simulink model "mOvertakeManeuver"  (R2018b)
settings: Solver=VariableStepAuto  StartTime=0.0  StopTime=simTime  RelTol=1e-3
PreLoadFcn:
  | load 'tableStructure.mat'
InitFcn:
  | modelParams
  | clear markedSmartActorCount;
values from neighbouring files (symbols this model uses):
  initYPos = (scene.RoadNetwork.RoadCenters(1, 2) - laneWidth / 2)    [modelParams.m]
  initYPosRogue = (scene.RoadNetwork.RoadCenters(1, 2) - laneWidth / 2)    [modelParams.m]
  laneWidth = roadWidth / (scene.RoadNetwork.NumMarkings - 1)    [modelParams.m]
  maxLanes = 10    [modelParams.m]
  maxVehicles = 25    [modelParams.m]
  minOvertakeProximity = 50    [modelParams.m]
  numActors = length(scene.vehiclePoses(1).ActorPoses)    [modelParams.m]    (also in sessionLogReader.m = numel(inStruct); visualizer.m = numel(actors))
  numAddedRogueActors = 0    [modelParams.m]
  numLanes = scene.RoadNetwork.NumLanes    [modelParams.m]    (also in sessionLogReader.m = numMarkings-1)
  numSmartActors = 0    [modelParams.m]
  numSmartActorsDM = 0    [modelParams.m]
  rogueActorIdBase = 4000    [modelParams.m]
  safeTimeGap = 1.4    [modelParams.m]
  sensorRange = 600    [modelParams.m]
  smartActors = 0    [modelParams.m]    (also in sessionLogReader.m = repmat(actorPoses(1), [obj.NumSmartActors, 1]))
  smartActorsDM = 0    [modelParams.m]    (also in sessionLogReader.m = repmat(actorPoses(1), [obj.NumSmartActorsDM, 1]))
  standStillGap = 10    [modelParams.m]
  W_SPEC = [Ln1;vdes;vmax;AXadd;AXmult;BXadd;BXmult;EXadd;EXmult;CXconst;CXadd;CXmult;OPDVmult;OPDVadd;BNULLmult;BMAXmult;FAKTORVmult;BMINadd;BMINmult;      RND1n;RND2n;RND3n;RND4n;NRND]    [wiedemannParams.m]
undefined symbols (not defined in the file or in its folder): actorPoseInit, addedRogueVelocity, addedRogueXPosition, DiscIntNeverNeededParam
libraries: dataTableBlockslib x2, mpcadaslib x1
(part 2 of 3)

== matlab function mOvertakeManeuver/Wiedemann-74 Driver Model/Apply driver-model/Extract InitPos and InitVel Vector ==
  data: accelVector input; smartActorsDM parameter; accelVector output; initVelVector output; initPosVector output; actorPoseInit parameter
function [accelVector, initVelVector, initPosVector] = extractInitPoses(accelVector, smartActorsDM, actorPoseInit)
% Extract init poses for vehicles with car-following model.
numActors = length(smartActorsDM);
initPosVector = ones(numActors,1);
initVelVector = ones(numActors,1);
for i = 1 : numActors
    initPosVector(i) = actorPoseInit(uint32(smartActorsDM(i))).Position(1);
    initVelVector(i) = actorPoseInit(uint32(smartActorsDM(i))).Velocity(1);
    if actorPoseInit(uint32(smartActorsDM(i))).Yaw == 180 % Actor is moving in negative - x dir
        accelVector(i) = -accelVector(i);
    end
end

== matlab function mOvertakeManeuver/Wiedemann-74 Driver Model/Apply driver-model/Wiedemann-driver-model/Judgement/Wiedemann74 ==
  data: xn input; bn output; vn input; xn1 input; vn1 input; bn1 input; regime output; AXAdd parameter; BXMult parameter; W_SPEC input; maxAccel parameter; maxDecel parameter; vMax parameter; vDes parameter
function [bn,regime] = wiedemann74(xn, vn, xn1, vn1, bn1, AXAdd, BXMult, W_SPEC, maxAccel, maxDecel, vMax, vDes)
% Wiedemann 74 car-following model
% input
% xn: ego vehicle position
% vn: ego vehicle velocity
% xn1: lead vehicle position
% vn1: lead vehicle velocity
% bn1: lead vehicle acceleration
% W_SPEC: model parameters
% output
% bn: ego vehicle acceleration command, i.e., driver's judgement
% regime: driver's operating mode
% (1 = following, 2 = free driving, 3 = approaching, 4 = emergency, -1 = danger)

numActors = size(xn, 1);
persistent dirAccel dx_old dv_old
if isempty(dirAccel)
    dirAccel = ones(numActors, 1);
end
if isempty(dx_old)
    dx_old = ones(numActors, 1);
    for i = 1 : numActors
        dx_old(i) = abs(xn1(i) - xn(i));
    end
end
if isempty(dv_old)
    dv_old = ones(numActors, 1);
    for i = 1 : numActors
        dv_old(i) = vn(i) - vn1(i);
    end
end

bn = ones(numActors, 1);
regime = ones(numActors, 1);
for i = 1 : numActors
    % variables
    dx = abs(xn1(i) - xn(i)); % [m] space headway
    dv = vn(i) - vn1(i); % [m/s] difference in speed
    % parameters
    % User-configured parameters
    AXadd = AXAdd(i);
    BXmult = BXMult(i);
    vmax = vMax(i);
    vdes = vDes(i);
    % Other parameters for which all the cars share the same value
    Ln1 = W_SPEC(1);
    AXmult = W_SPEC(5);
    BXadd = W_SPEC(6);
    EXadd = W_SPEC(8);
    EXmult = W_SPEC(9);
    CXconst = W_SPEC(10);
    CXadd = W_SPEC(11);
    CXmult = W_SPEC(12);
    OPDVmult = W_SPEC(13);
    OPDVadd = W_SPEC(14);
    BNULLmult = W_SPEC(15);
    BMAXmult = 3.5 / vmax;
    FAKTORVmult = W_SPEC(17);
    BMINadd = W_SPEC(18);
    BMINmult =  1.5 / vmax;
    RND1n = W_SPEC(20);
    RND2n = W_SPEC(21);
    RND3n = W_SPEC(22);
    RND4n = W_SPEC(23);
    NRND = W_SPEC(24);
    
    % threshold of driver's operating regime
    % AX: Minimum distance headway (front-bumper to front-bumper distance) in a standstill condition
    AX = Ln1 + AXadd + AXmult * RND1n;
    
    % ABX: Minimum desired following distance
    v_slower = min(vn(i), vn1(i));
    BX = (BXadd + BXmult * RND1n) * sqrt(v_slower);
    ABX = AX + BX;
    
    % SDX: Maximum desired following distance
    EX = EXadd + EXmult * (NRND - RND2n);
    SDX = AX + EX * BX;
    
    % SDV: Threshold at which driver recognizes that he is approaching a slower vehicle
    CX = CXconst * (CXadd + CXmult * (RND1n + RND2n));
    SDV = ((dx - Ln1 - AX) / CX)^2;
    
    % CLDV: Threshold for speed difference in a closing process during a following condition
    CLDV = SDV; % CLDV is assumed to be equal to SDV
    
    % OPDV: Threshold for speed difference in an opening process during a following condition
    OPDV = CLDV * (-OPDVadd - OPDVmult * NRND);
    
    % acceleration/deceleration command
    if (dx >= ABX) && (dv >= OPDV) && (dx <= SDX) && (dv <= SDV) % following
        if (SDV < dv_old(i)) || (dx_old(i) < ABX) % passing SDV, ABX
            dirAccel(i) = -1;
        elseif (dv_old(i) < OPDV) || (SDX < dx_old(i)) % passing OPDV, SDX
            dirAccel(i) = 1;
        end
        bnull = BNULLmult * (RND4n + NRND);
        bn(i) = dirAccel(i) * bnull;
        regime(i) = 1;
    elseif ((dx > ABX) && (dv < OPDV)) || ((dx > SDX) && (dv < SDV)) % free driving
        FaktorV = vmax / (vdes + FAKTORVmult * (vmax - vdes));
        bmax = BMAXmult * (vmax - v_slower * FaktorV);
        bn(i) = bmax;
        regime(i) = 2;
    elseif (dv > SDV) && (dx > ABX) % approaching
        bn(i) = 0.5 * dv^2 / (ABX - (dx - Ln1)) + bn1(i);
        regime(i) = 3;
    elseif (dx > AX) && (dx < ABX) % emergency
        bmin = -BMINadd - BMINmult * RND3n + BMINmult * vn(i);
        bn(i) = 0.5 * dv^2 / (ABX - (dx - Ln1)) + bn1(i) + bmin * (ABX - (dx - Ln1)) / BX;
        regime(i) = 4;
    else % danger
        bn(i) = 0;
        regime(i) = -1;
    end
    
    if(bn(i) > maxAccel(i)) % Limiting output accel/decel by upper and lower bounds
        bn(i) = maxAccel(i);
    elseif(bn(i) < maxDecel(i))
        bn(i) = maxDecel(i);
    end
    
    if(bn(i) < 0 && vn(i) < 0) % Not allowing backward-movement
        bn(i) = 0;
    end
    
    dv_old(i) = dv;
    dx_old(i) = dx;
end

== matlab function mOvertakeManeuver/Wiedemann-74 Driver Model/Get Follow and Lead car ==
  data: follPos output; follVel output; leadPos output double; leadVel output double; smartActorsDM parameter; leadAcc output; sensorRange parameter; timestamp input
function [follPos, follVel, leadPos, leadVel, leadAcc] = extractFollowAndLeadCar(...
    smartActorsDM, sensorRange, timestamp)
% For the cars with driver model, extract their info as well as their
% respective lead car info from the data-table.

% To store the current timestamp and velocity of respective
% lead vehicles for calculation of their acceleration in the next step.
% Also, as acceleration calculation requires velocity at two timestamps,
% 3rd column in this information has the flag indicating whether previous
% velocity info is available.
persistent prevInfo;
if(isempty(prevInfo))
    prevInfo = zeros(length(smartActorsDM), 3);
end

leadPos = ones(length(smartActorsDM), 1);
leadVel = ones(length(smartActorsDM), 1);
follPos = ones(length(smartActorsDM), 1);
follVel = ones(length(smartActorsDM), 1);
leadAcc = zeros(length(smartActorsDM), 1);

for i = 1 : length(smartActorsDM)
    key = getActorTableEntryKey(uint32(1), smartActorsDM(i));
    if(key ~= -1) % If an entry exist
        smartVehInfo = getActorTableEntry(key);
        [numVehAhead, vehiclesAheadInfo] = getVehAheadSorted(key);
        if(numVehAhead == 0)
            % There is no vehicle ahead of this smart vehicle
            % Give impression that vehicle ahead is out of sensor range
            if smartVehInfo.Velocity(1) < 0
                leadPos(i) = smartVehInfo.Position(1) - sensorRange;
            else
                leadPos(i) = smartVehInfo.Position(1) + sensorRange;
            end
            leadVel(i) = smartVehInfo.Velocity(1);
            leadAcc(i) = 0;
            prevInfo(i, 3) = 0;
        else
            leadPos(i) = vehiclesAheadInfo(1).Position(1); % Get position of vehicle just ahead.
            leadVel(i) = vehiclesAheadInfo(1).Velocity(1); % Get speed of vehicle just ahead.
            if(prevInfo(i, 3) == 1) % If previous velocity known for accel calculation
                leadAcc(i) = (vehiclesAheadInfo(1).Velocity(1) - prevInfo(i, 2)) / ...
                    (timestamp - prevInfo(i, 1));
            else
                leadAcc(i) = 0 ;
            end
        end
        follPos(i) = smartVehInfo.Position(1);
        follVel(i) = smartVehInfo.Velocity(1);
        prevInfo(i, 1) = timestamp;
        prevInfo(i, 2) = vehiclesAheadInfo(1).Velocity(1);
        prevInfo(i, 3) = 1; % Acceleration can be calculated at next time-step.
        leadVel(i) = abs(leadVel(i));
        follVel(i) = abs(follVel(i));
        if smartVehInfo.Yaw == 180 % Actor is moving in negative - x dir
            leadAcc(i) = -leadAcc(i);
        end
    end
end

== matlab function mOvertakeManeuver/Services/Find approaching vehicles in the left lane/MATLAB Function ==
  data: refPose input; matched output; candidatePose input; sensorRange parameter; laneWidth parameter; numLanes parameter
function matched = findVehiclesAheadLeftLane(refPose, candidatePose, sensorRange, laneWidth, numLanes)
% For any vehicle, get the vehicles ahead in the opposite lane. Query is
% assumed to called for a vehicle moving in +ve x-direction.
% refVeh - Query-Calling vehicle
% candidateVeh - Actor to be processed as candidate for matching the criteria.

laneBoundaries = zeros(1, numLanes + 1);
% Getting the key corresponding to the actorId from data-table
key = getScenarioTableEntryKey(uint32(1), refPose.ActorID);
completeLaneBoundaryInfo = getScenarioTableEntry(key);
for i = 1 : size(laneBoundaries, 2)
    laneBoundaries(1, i) = completeLaneBoundaryInfo.coordinates(i, 2);
end
laneIndx = -1;
% Find own lane information based on lane boundary info and own pose info.
for i = 1 : size(laneBoundaries, 2) - 1
    if (refPose.Position(2) <= laneBoundaries(1, i) && refPose.Position(2) >= laneBoundaries(1, (i + 1)))
        laneIndx = i;
        break;
    end
end
if laneIndx < 0
    matched = false;
elseif laneIndx <= numLanes
    xGap = (candidatePose.Position(1) - refPose.Position(1));
    yGap = (candidatePose.Position(2) - refPose.Position(2));
    gap = sqrt(xGap * xGap + yGap * yGap);
    
    % Candidate actor must be ahead AND in Range AND In opposite(left) lane
    if ((xGap > 0)  && gap < sensorRange && ((candidatePose.Position(2) >= laneBoundaries(1, laneIndx))) ...
            && ((candidatePose.Position(2) <= (laneBoundaries(1, laneIndx) +  laneWidth))))
        matched = true;
    else
        matched = false;
    end
else
    matched = false;
end

== matlab function mOvertakeManeuver/Scene Management/Publish To Data Table/update data tables ==
  data: actors input; laneBoundaryInfo input; maxLanes parameter; smartActorsDM parameter; smartActors parameter
function updateDataTables(actors, laneBoundaryInfo, maxLanes, smartActorsDM, smartActors)
% Write into actor-pose table and scene table(containing lane boundary information)

% Write into actor-pose table
for k = 1 : length(actors)
    % Write the actor-poses into the data-table (Except for the smart
    % actors to avoid re-writing in the data-table the same data which we just read)
    if ~(ismember(actors(k).ActorID, smartActors) || ismember(actors(k).ActorID, smartActorsDM))
        setActorTableEntry(actors(k).ActorID, actors(k)); % Use key to update the row entry.
    end
end

% Write lane boundary information of smart actors into scene data-table.
numLanes = laneBoundaryInfo.NumLaneBoundaries;
for i = 1 : length(laneBoundaryInfo.ActorIDs)
    laneBoundary.ActorID = laneBoundaryInfo.ActorIDs(i);
    laneBoundary.coordinates = ones(maxLanes, 3) * (double(intmax('uint32')));
    for j = 1 : numLanes % For each lane writing x,y,z coordinates
        for k = 1 : 3 % For x,y and z
            laneBoundary.coordinates(j, k) = laneBoundaryInfo.LaneBoundaries(i, j).Coordinates(1, k);
        end
    end
    setScenarioTableEntry(laneBoundary.ActorID, laneBoundary); % Write into scene data-table.
end

== stateflow chart mOvertakeManeuver/Smart Actor/Smart Actor system/Planner/Plan Library and its evaluation/Plan 1/Plan 1: Overtake Maneuver/checkOvertakeFeasibility/Check feasibilty of the overtake ==
  note: Algorithm to decide if in the current environment, smart-car can start an overtake-maneuver right away.
      | It does so by anticipating movement of other vehicles and its own trajectory for overtake maneuver.
      |
      | Note: The overtake maneuver plan assumes that all other actors move straight with constant speed.
      |
      | Structure of this chart is such, that it sequentially does various checks for ensuring that overtake mauver is safe.Whenever any check fails the overtake is deemed as unsafe. Only when all the conditions meet, the chart returns 'overtakeDecision=1' (which happens at the bottom-right of chart after passing all the tests).
  (default) -> (junction 615) : {
      | actorStruct = struct('ActorID',double(intmax('uint32')), 'Position', [0 0 0], ...
      |                       'Velocity', [0 0 0], 'Roll', 0, 'Pitch', 0, 'Yaw', 0, ...
      |                       'AngularVelocity', [0 0 0]);
      |
      | % Variables initialization
      | vehiclesAheadList = repmat(actorStruct, maxVehicles, 1);
      | rogueOppDir  = repmat(actorStruct, maxVehicles, 1);
      | overtakeDecision = 0;
      | t1 = 0;  % Time spent for moving towards opposite direction lane.
      | t2 = 0;  % Time spent for moving in opposite direction lane.
      | t3 = 0;  % Time spent for merging back into original lane
      |
      | % Value = 1 if smart vehicle is going to merge between 2 vehicles after overtake.
      | % Value = 0 if smart vehicle would not have a vehicle ahead after overtake.
      | mergeBehindVehFlag = 0;
      |
      | leftLaneCenter = getLeftLane(currPose);
      | precedVehInfo = actorStruct;
      | }
  (junction 615) -> (junction 616) [order 1] : % If left lane present
      | [leftLaneCenter ~= realmax('double') ]
  (junction 615) -> (junction 660) [order 2] : {
      | % No lane on the left where smart-vehicle
      | % can move temporarily for overtake
      | overtakeDecision = 0;
      | }
  (junction 616) -> (junction 713) : {
      | leftLaneChangeDistY = leftLaneCenter - currPose.Position(2);
      |  % Assuming 45 deg movement towards adjacent lane
      | leftLaneChangeDistance =  leftLaneChangeDistY * 1.414;
      | rightLaneChangeDistance  = laneWidth * 1.414;
      | smartActorPosition = currPose.Position;
      |
      | % Get list of vehicles ahead moving in the same lane in sorted
      | % order of their distance from smart vehicle.
      | [count, vehiclesAheadList] = getVehAheadSameLaneSorted(currPose);
      |
      | % Set the limit on number of vehicles allowed to be overtaken
      | % in a single go based on driver aggresiveness level.
      | maxOvertakeCapability =  aggressivenessLevel;
      | i=1;
      | }
  (junction 713) -> (junction 709) [order 1] : [i<=count]
  (junction 710) -> (junction 713) : {
      |      i=i+1;
      | }
  (junction 713) -> (junction 467) [order 2]
  (junction 709) -> (junction 710) : {
      |     % Convert to self-centered pose
      |      vehiclesAheadList(i) = ...
      |      globalToSelfCentered(currPose, vehiclesAheadList(i));
      | }
  (junction 467) -> (junction 660) [order 2] : {
      | % No vehicle ahead to overtake
      | overtakeDecision = 0;
      | }
  (junction 467) -> (junction 469) [order 1] : [count > 0  ]
  (junction 660) -> (junction 663)
  (junction 469) -> (junction 471) : {
      | % Get vehicle just ahead
      | nearestVehInfo = vehiclesAheadList(1);
      | }
  (junction 471) -> (junction 663) [order 2] : {
      | % Vehicle ahead is too far so no need to overtake
      | overtakeDecision = 0;
      | }
  (junction 471) -> (junction 473) [order 1] : % Vehicle ahead must be close enough
      | % to initiate overtake
      |   [nearestVehInfo.Position(1) < ...
      |    minOvertakeProximity]
  (junction 663) -> (junction 666)
  (junction 473) -> (junction 27)
  (junction 27) -> (junction 47) [order 1] : [count < maxOvertakeCapability]
  (junction 27) -> (junction 48) [order 2] : {
      |      overtakeLen = maxOvertakeCapability;
      | }
  (junction 47) -> (junction 49) : {
      |     overtakeLen = count ;
      | }
  (junction 49) -> (junction 48)
  (junction 48) -> (junction 70)
  (junction 70) -> (junction 666) [order 2] : {
      | % No possibility of overtake-maneuver.
      | % All possibilities right from max-capability
      | % overtake to 1-vehicle-overtake are checked
      | % but none was feasible.
      | overtakeDecision = 0;
      | }
  (junction 70) -> (junction 69) [order 1] : % Loop through all possible overtake maneuvers.
      | %Start feasibilty check from maximum length overtake upto 1-vehicle-overtake
      | % and exit the loop whenever first feasibility check is successful
      | [overtakeLen > 0]
  (junction 666) -> (junction 264)
  (junction 682) -> (junction 70) : {
      | % Decrement for 1-lesser level overtake
      | overtakeLen = overtakeLen - 1;
      | }
  (junction 69) -> (junction 621) : {
      |     % Vehicle to be checked for overtaking
      |     followVehInfo = vehiclesAheadList(overtakeLen);
      | }
  (junction 621) -> (junction 682) [order 2] : % Cannot overtake a vehicle moving
      | % at a higher speed than this (smart) vehicle's
      | % max speed.
      | % Check for 1-lesser level overtake
  (junction 621) -> (junction 73) [order 1] : % Overtake possible only if vehicle ahead is moving at
      |  % lesser speed than smart actor's max speed.
      |  [maxVelocity >  ...
      | (followVehInfo.Velocity(1) + currPose.Velocity(1)) ...
      | && currPose.Velocity(1) > 0]
  (junction 73) -> (junction 81) [order 1] : [overtakeLen < count]
  (junction 685) -> (junction 682)
  (junction 73) -> (junction 96) [order 2]
  (junction 81) -> (junction 92) : {      % Vehicle Id to be checked for merging behind
      |         % Smart vehicle is cheking possiblity of merging between actors
      |         % having pose 'followVehInfo' and 'precedVehInfo'
      |         mergeBehindVehFlag = 1;
      | 	  precedVehInfo = vehiclesAheadList(overtakeLen + 1);
      |         reqSafeGap = 2 * ((currPose.Velocity(1) + precedVehInfo.Velocity(1)) ...
      |                                * safeTimeGap + standStillGap);
      |         gap = precedVehInfo.Position(1) - followVehInfo.Position(1);
      | }
  (junction 92) -> (junction 685) [order 2] : % Not enough gap present between two vehicles
      | % for merging in between after overtake maneuver
      | % Check for 1-lesser level overtake
  (junction 92) -> (junction 93) [order 1] : % Not enough gap between vehicles in smart actor's
      | % lane to merge in between after overtaking.
      | [gap >= reqSafeGap]
  (junction 669) -> (junction 685)
  (junction 93) -> (junction 94)
  (junction 94) -> (junction 96)
  (junction 96) -> (junction 608) : {
      |     [t1, smartVehXT1, t2, smartVehXT2, t3, smartVehXT3, smartVehSpeedT3] =  ...
      |     anticipateManeuverSubTrajectories();
      |
      |     T = t1 + t2 +t3; % Total time taken for overtake maneuver
      |     }
  (junction 608) -> (junction 483) : {
      |    % Need to check safety w.r.t vehicle coming from opposite direction
      |     oppositeDirSafety = anticipateOppositeDirTrafficSafety();
      | }
  (junction 483) -> (junction 669) [order 2] : % Not safe w.r.t oppsite direction traffic
      | % Check for 1-lesser level overtake
  (junction 483) -> (junction 185) [order 1] : [oppositeDirSafety==1]
  (junction 678) -> (junction 669)
  (junction 185) -> (junction 245) : {
      |     isSafeAfterOvertake =  ...
      |     anticipateSafetyAfterManeuverCompletion(smartVehXT3);
      | }
  (junction 245) -> (junction 678) [order 2] : %  Not safe w.r.t. to vehicles it is planning
      | % to merge in between after overtake.
      | % Check for 1-lesser level overtake
  (junction 245) -> (junction 672) [order 1] : [isSafeAfterOvertake==1]
  (junction 672) -> (junction 192)
  (junction 192) -> (junction 264) : {
      | % All conditions met for safe overtake.
      | overtakeDecision = 1;
      | }
  (junction 264) -> (junction 688)
  data: time1 function_output; smartXPos1 function_output; time2 function_output; smartXPos2 function_output; time3 function_output; smartXPos3 function_output; smartXVel3 function_output; isSafe function_output; isSafe function_output; smartXPosT3 function_input; overtakeDecision output; currPose input Bus: Vehicle; maxVelocity parameter; maxAcceleration parameter; nearestVehInfo local Bus: Vehicle; safeTimeGap parameter; standStillGap parameter; followVehXT2 local; followVehspeedT2 local; leftLaneChangeDistY local; rightLaneChangeDistance local; T local; a local; b local; c local; count local; d local; smartActorPosition local; smartVehXT1 local; smartVehXT2 local; followVehSpeed local; followVehXT1 local; gap local; gapBack local =0; gapFront local =0; leadRogueOppDirInfo local Bus: Vehicle; leadRogueOppDirPos local =0; leftLaneChangeDistance local; mergeBehindVehFlag local; oppRogueCount local; overtakeLen local; reqSafeGap local; reqSafeGapBack local =0; reqSafeGapFront local =0; rogueOppDir local Bus: Vehicle; s2 local; s21 local; t21 local; t22 local; vehiclesAheadList local Bus: Vehicle; smartVehSpeedT3 local; followVehXT3 local =0; smartVehXT3 local; pPrecedingRogue local =0; vehicleAheadOvertakenRogueDetails local Bus: Vehicle; laneWidth parameter; actorStruct local Bus: Vehicle; maxOvertakeCapability local; precedVehInfo local Bus: Vehicle; followVehInfo local Bus: Vehicle; i local; t1 local; t3 local; t2 output; d1 local; d2 local; t23 local; safeGapDeficit local; maxVehicles parameter; minOvertakeProximity parameter; leftLaneCenter local; oppositeDirSafety local; isSafeAfterOvertake local; aggressivenessLevel parameter
  function [time1, smartXPos1, time2, smartXPos2, time3, smartXPos3, smartXVel3] = anticipateManeuverSubTrajectories:
    | function [time1, smartXPos1, time2, smartXPos2, time3, smartXPos3, smartXVel3] = anticipateManeuverSubTrajectories()
    | % Anticipate smart-actors sub-trajectories for overtake-maneuver trajectory.
    | % time1 - Time soent in sub-trajectory 1 ( i.e. Movement towards left lane)
    | % smartXPos1 - Smart actor's X-pos at the end of sub-trajectory 1
    | % time2 - Time soent in sub-trajectory 2 ( i.e. Movement on the left lane)
    | % smartXPos2 - Smart actor's X-pos at the end of sub-trajectory 2
    | % time3 - Time soent in sub-trajectory 3 ( i.e. Movement back to original lane)
    | % smartXPos3 - Smart actor's X-pos at the end of sub-trajectory 3
    | % smartXVel3 - Smart actor's X-vel at the end of sub-trajectory 3
    | 
    | % Calculate the time to reach the adjacent lane
    | time1 = leftLaneChangeDistance / currPose.Velocity(1) ;
    | 
    | % Anticipated position and velocity of smart Veh and 'followVehId' after
    | % 'time1' time units after overtake maneuver start i.e the time after which
    | % smart vehicle reaches the adjacent lane.
    | % Note: This is just anticipated information. Vehicles move in real only if
    | % overtake maneuver turn out to be safe in the logic below.
    | smartXPos1 =   currPose.Position(1) + leftLaneChangeDistance;
    | followVehXT1 =  (currPose.Position(1) + followVehInfo.Position(1)) + ...
    |     (currPose.Velocity(1) + followVehInfo.Velocity(1)) * time1;
    | smartVehSpeedT1 = currPose.Velocity(1);
    | followVehSpeed = currPose.Velocity(1) + followVehInfo.Velocity(1);
    | 
    | % Anticipitation of position and velocity info after t = time1+time2.
    | % 'time2' is the time elapsed from the point smart vehicle reached adjacent
    | % lane upto the time after which smart vehicle has accumulated safe gap with
    | % respect to the vehicle to be overtaken while moving parallel to it in the
    | % adjacent lane. This condition when used with Newton's equations of motion
    | % results into a quadratic equation of form ax2+bx+c where x='time2' and
    | % a,b,c defined below.
    | a = 0.5 * maxAcceleration;
    | b = smartVehSpeedT1 - followVehSpeed;
    | c = smartXPos1 - followVehXT1 - followVehSpeed * safeTimeGap - standStillGap;
    | d = (b ^ 2) - (4 * a * c);
    | time2a = (- b + sqrt(d)) / (2 * a); % first root of equation
    | time2b = (- b - sqrt(d)) / (2 * a); % second root of equation
    | if(time2a > 0) % Only positive root is meaningful
    |     time2 = time2a;
    | else
    |     time2 = time2b;
    | end
    | 
    | smartVehSpeedT2 = smartVehSpeedT1 + maxAcceleration * time2; % Speed of smart vehicle after time1 + time2
    | s2 = smartVehSpeedT1 * time2 + 0.5 * maxAcceleration * time2 ^ 2;
    | 
    | if(smartVehSpeedT2 > maxVelocity)
    |     % After time time2 smart vehicle is going to breach
    |     % max velocity allowed, so time time2 is broken into time2a and time2b .
    |     % time2a - time to reach max vel
    |     % time2b - time to accumulate safe gap w.r.t vehicle being overtaken after reaching max velocity
    |     
    |     % Distance travelled in the process of reaching max velocity.
    |     s21 = ((maxVelocity ^ 2) - (smartVehSpeedT1 ^ 2)) / (2 * maxAcceleration);
    |     t21 = (maxVelocity - smartVehSpeedT1) / maxAcceleration;
    |     t22 = ((followVehSpeed * safeTimeGap + standStillGap) - (smartXPos1 + s21) + ...
    |         (followVehXT1 + followVehSpeed * t21)) / (maxVelocity - followVehSpeed);
    |     % Total time travelled by the smart car in adjacent lane to create safeGap between the the rogue car and itself
    |     time2 = t21 + t22;
    |     smartVehSpeedT2 = maxVelocity;
    |     s2 = s21 + maxVelocity * t22 ;
    | end
    | 
    | smartXPos2 = smartXPos1 + s2  ;
    | followVehXT2 = followVehXT1 + followVehSpeed * time2;
    | followVehspeedT2 = followVehSpeed;
    | %total time after which merging into the actual lane will be started
    | T =  time1 + time2 ;
    | 
    | time3 = rightLaneChangeDistance / smartVehSpeedT2;
    | d1 = laneWidth;
    | d2 = followVehspeedT2 * time3;
    | 
    | if(d1 < d2)
    |     safeGapDeficit = d2 - d1;
    |     t23 = safeGapDeficit / (smartVehSpeedT2 - followVehspeedT2);
    |     smartXPos2 = smartXPos2 + smartVehSpeedT2 * t23 ;
    |     followVehXT2 = followVehXT2 + followVehspeedT2 * t23;
    |     T =  T + t23;
    | end
    | 
    | % time3 is the time taken by smart vehicle to again move to its original lane
    | % after it has accumulated safe gap w.r.t to vehicle to be
    | % overtaken. Safety condition at this time is that after merging into the
    | % main lane smart vehicle shouldbe safe wrt the vehicles it is merging
    | % between.
    | 
    | time3 = rightLaneChangeDistance / smartVehSpeedT2;
    | smartXPos3 = smartXPos2 + rightLaneChangeDistance;
    | smartXVel3 = smartVehSpeedT2;
  function isSafe = anticipateOppositeDirTrafficSafety:
    | function isSafe = anticipateOppositeDirTrafficSafety
    | % Anticipate whether smart-actor is safe w.r.t to traffic from opposite
    | % direction for overtake maneuver.
    | 
    | isSafe = 1;
    | % Find the rogue vehicles approaching from the opposite direction
    | [oppRogueCount, rogueOppDir]  = getVehAheadLeftLaneSorted(currPose);
    | for i=1:oppRogueCount % Convert to self-centered pose
    |     rogueOppDir(i) = globalToSelfCentered(currPose, rogueOppDir(i));
    | end
    | i = 1;
    | % For each rogue veh from the opposite direction, check safety.
    | for i = 1 : oppRogueCount
    |     leadRogueOppDirInfo = rogueOppDir(i);
    |     % Its anticipated position after end of subTrajectory-2 i.e after it
    |     % has finished movement on opposite direction lane.
    |     leadRogueOppDirPos = leadRogueOppDirInfo.Position(1) + smartActorPosition(1) ...
    |         + ((leadRogueOppDirInfo.Velocity(1) +  currPose.Velocity(1)) * T);
    |     % Anticipated gap between this and smart vehicle after time = t1 + t2
    |     gap = leadRogueOppDirPos - smartVehXT2 ;
    |     
    |     % Smart actor must not collide or be in unsafe proximity of actor coming from
    |     % opposite direction
    |     if(gap <= 2 * standStillGap)
    |         isSafe = 0; % Not safe
    |         break;
    |     end
    | end
  function isSafe = anticipateSafetyAfterManeuverCompletion (smartXPosT3):
    | function isSafe = anticipateSafetyAfterManeuverCompletion (smartXPosT3)
    | % Anticipate whether smart-actor is safe after it merges back to its original
    | % lane i.e. after completion of overtake maneuver. Basically at that point
    | % smart actor must be safe w.r.t vehicles it is merging in between.
    | 
    | isSafe = 1;
    | followVehSpeed = currPose.Velocity(1) + followVehInfo.Velocity(1);
    | followVehXT1 =  (currPose.Position(1) + followVehInfo.Position(1)) + ...
    |     (currPose.Velocity(1) + followVehInfo.Velocity(1)) * t1;
    | followVehXT2 = followVehXT1 + followVehSpeed * t2;
    | 
    | followVehXT3 = followVehXT2 + followVehSpeed * t3;
    | 
    | vehicleAheadOvertakenRogueDetails = precedVehInfo;
    | reqSafeGapFront =  smartVehSpeedT3  * safeTimeGap + standStillGap;
    | reqSafeGapBack = followVehSpeed * safeTimeGap + standStillGap;
    | pPrecedingRogue = vehicleAheadOvertakenRogueDetails.Position(1) + currPose.Position(1) +  ...
    |     (currPose.Velocity(1) + vehicleAheadOvertakenRogueDetails.Velocity(1)) * T;
    | gapFront =  pPrecedingRogue - smartXPosT3;
    | gapBack =  smartXPosT3 - followVehXT3;
    | 
    | % If there a vehicle ahead after manaeuver then the smart vehicle needs to
    | % check both front and back safety. Otherwise smart vehicle just needs to be
    | % safe with respect to vehicle it is merging ahead of, after overtake.
    | if(mergeBehindVehFlag)
    |     if (gapFront < reqSafeGapFront || gapBack < reqSafeGapBack)
    |         isSafe = 0; % Not safe
    |     end
    | else
    |     if(gapBack < reqSafeGapBack)
    |         isSafe = 0; % Not safe
    |     end
    | end

== matlab function mOvertakeManeuver/Services/Global to self-centered pose conversion/Self-Centered Pose Conversion ==
  data: selfPose input; otherVehPose input Bus: Vehicle; egoCentricInfo output Bus: Vehicle
function egoCentricInfo = globalToSelfCenteredConversion(selfPose, otherVehPose)
% Convert global-coordinate pose of another vehicle to self-centered pose.

egoCentricInfo.ActorID = otherVehPose.ActorID;
egoCentricInfo.Position = otherVehPose.Position - selfPose.Position;
egoCentricInfo.Velocity = otherVehPose.Velocity - selfPose.Velocity;
egoCentricInfo.Roll = otherVehPose.Roll - selfPose.Roll;
egoCentricInfo.Pitch = otherVehPose.Pitch - selfPose.Pitch;
egoCentricInfo.Yaw = otherVehPose.Yaw - selfPose.Yaw;
egoCentricInfo.AngularVelocity = otherVehPose.AngularVelocity - selfPose.AngularVelocity;

== matlab function mOvertakeManeuver/Wiedemann-74 Driver Model/Write smart-actor poses in data-table ==
  data: smartActorsDM parameter; velVector input; posVector input
function updateSmartCarPose(smartActorsDM, velVector, posVector)
% Update the Pose value of the vehicles having car-following model with
% those calculated using Wiedemann-74 driver model.

numActors = length(smartActorsDM);
for i = 1 : numActors
    % Retrieve the key based on passed Actor ID value
    % Note: As Actor ID is first field in the entry the field index is
    % passed as 1
    key = getActorTableEntryKey(uint32(1), smartActorsDM(i));
    if(key ~= -1) % If an entry exist
        actorInfo = getActorTableEntry(key);
        actorInfo.Position(1) = posVector(i);
        actorInfo.Velocity(1) = velVector(i);
        setActorTableEntry(key, actorInfo);
    end
end

== matlab function mOvertakeManeuver/Wiedemann-74 Driver Model/Gets the vehicles ahead in sorted order of the distance from this actor./Gets the vehicles ahead in sorted order of the gap ==
  data: actorId input; vehAheadInfo output Bus: Vehicle size=maxVehicles; numVeh output; maxVehicles parameter
function [vehAheadInfo, numVeh]  = getVehAheadSorted(actorId, maxVehicles)
% Returns the list of vehicle ahead in sorted order of the gap from the query-calling vehicle.

y.ActorID = double(intmax('uint32'));
y.Position = [0 0 0];
y.Velocity = [0 0 0];
y.Roll = 0;
y.Pitch = 0;
y.Yaw = 0;
y.AngularVelocity = [0 0 0];
vehAheadInfo = repmat(y, maxVehicles, 1);
actorId = double(actorId);
smartVehInfo = getActorTableEntry(actorId);
qHdl = initActorQueryIterator(actorId, uint32(OvertakeQueries.VehiclesAheadSameLane));
[key, done] = getActorQueryIterNextKey(qHdl);
mIdx = 1;
% Get next vehicle-of-interest and put in a sorted way according to its
% distance from this actor
while ~done
    info = getActorTableEntry(key);
    if(mIdx == 1) % First vehicle
        vehAheadInfo(mIdx) = info;
    else
        i = (mIdx - 1);
        if smartVehInfo.Yaw == 0 % Positive - x
            while(i >= 1 && (info.Position(1) < vehAheadInfo(i).Position(1)))
                % Insert at correct place to maintain sorted order
                vehAheadInfo(i + 1) = vehAheadInfo(i);
                i = i - 1;
            end
            vehAheadInfo(i + 1) = info;
        elseif smartVehInfo.Yaw == 180 % Negative - x
            while(i >= 1 && (info.Position(1) > vehAheadInfo(i).Position(1)))
                % Insert at correct place to maintain sorted order
                vehAheadInfo(i + 1) = vehAheadInfo(i);
                i = i - 1;
            end
            vehAheadInfo(i + 1) = info;
        else
            % No direction
        end
    end
    mIdx = mIdx + 1;
    [key, done] = getActorQueryIterNextKey(qHdl);
end
numVeh = mIdx - 1;

== matlab function mOvertakeManeuver/Scene Management/Actor Pose Reader/Read smart actor poses ==
  data: numSmartActors parameter; smartActors parameter; numSmartActorsDM parameter; smartActorsDM parameter; actorPoseInit parameter Bus: Vehicle; initYPos parameter; actorPoses output Bus: Vehicle
function actorPoses = getSmartActorPose(numSmartActors, smartActors, numSmartActorsDM, ...
    smartActorsDM, actorPoseInit, initYPos)
% Read poses of all the smart actors ( i.e. regular-smart-actors and
% smart-actors-with-driver-model) from the data-table

% actorPoses - Poses of all smart actors.

% numSmartActors - Number of actors marked as smart.
% smartActors - Ids of actors marked as smart.
% numSmartActorsDM - Number of actors with driver model installed
% smartActorsDM - Ids of actors with driver model installed
% actorPoseInit - Initial pose information of session-log actors.

actorStruct = struct('ActorID', 0, 'Position', [0 0 0], ...
    'Velocity', [0 0 0], 'Roll', 0, 'Pitch', 0, 'Yaw', 0, ...
    'AngularVelocity', [0 0 0]);
% Create an actor structure array for all required actors
smartPoses = repmat(actorStruct, [numSmartActors, 1]);
smartPosesDM = repmat(actorStruct, [numSmartActorsDM, 1]);

% Read updated smart-actors poses from the data-table
for i = 1 : numSmartActors
    % Getting the key corresponding to the actor Id from the data table
    % As Actor ID is first field in the entry the field index is
    % passed as 1
    key = getActorTableEntryKey(uint32(1), smartActors(i));
    if (key ~= -1) % Retrieve the actor details based on key
        smartPoses(i) = getActorTableEntry(key);
    else % No entry yet with 'actor ID = smartActors(i)' in data-table
        smartPoses(i) = actorPoseInit(smartActors(i));
        smartPoses(i).Position(2) = initYPos;
        smartPoses(i).Yaw = 0;
    end
end

% Read updated smart-actors-DM(Actors with driver model installed) poses from the
% data-table
for i = 1 : numSmartActorsDM
    % Getting the key corresponding to the actorId from the data table
    % As Actor ID is first field in the entry the field index is
    % passed as 1
    key = getActorTableEntryKey(uint32(1), smartActorsDM(i));
    if key ~= -1
        % Retrieve the actor details based on key
        smartPosesDM(i) = getActorTableEntry(key);
    else % No entry yet with 'actor ID = smartActorsDM(i)' in data-table
        smartPosesDM(i) = actorPoseInit(smartActorsDM(i));
    end
end

% Concatenate the poses of smart actors and smart actors with driver model
% to return a combined bus.
actorPoses = [smartPoses; smartPosesDM];

== matlab function mOvertakeManeuver/Smart Actor/Smart Actor system/Find center of my left lane/Get left lane center Y ==
  data: currPose input; leftlaneY output; numLanes parameter
function leftlaneY = getLeftLaneY(currPose, numLanes)
% Get the Y-Coordinate of the left lane center

laneBoundaries = zeros(1, numLanes + 1);
% Getting the key corresponding to the actorId from data-table
key = getScenarioTableEntryKey(uint32(1), currPose.ActorID);
completeLaneBoundaryInfo = getScenarioTableEntry(key);
for i = 1 : size(laneBoundaries, 2)
    laneBoundaries(1, i) = completeLaneBoundaryInfo.coordinates(i, 2);
end
index = 0;
% Search the left lane based on the current position
for i = 1 : size(laneBoundaries, 2) - 1
    if (currPose.Position(2) <= laneBoundaries(1, i) && currPose.Position(2) >= laneBoundaries(1, (i + 1)))
        index = i;
        break;
    end
end
if (index > 1)
    leftlaneY = (laneBoundaries(1, index) + laneBoundaries(1, (index - 1))) / 2;
else
    % No left Lane present
    leftlaneY = realmax('double');
end

== matlab function mOvertakeManeuver/Scene Management/Append poses of added rouge actors for visualization/Appending Rouge Actor Poses ==
  data: Actors output Bus: Vehicle; numAddedRogueActors parameter; rogueActorIdBase parameter; simulationLogActors input
function Actors = appendRougeActorPoses(numAddedRogueActors, rogueActorIdBase, simulationLogActors)
% Create and output complete actor-pose stream by appending poses of
% additionally introduced rogue actors to the pose-stream of
% simulation-log actors.
actorStruct = struct('ActorID', 0, 'Position', [0 0 0], ...
    'Velocity', [0 0 0], 'Roll', 0, 'Pitch', 0, 'Yaw', 0, ...
    'AngularVelocity', [0 0 0]);
addedRogueActors = repmat(actorStruct, [numAddedRogueActors, 1]);
for i=1:numAddedRogueActors
    key = getActorTableEntryKey(uint32(1), (rogueActorIdBase + i));
    addedRogueActors(i) = getActorTableEntry(key);
end
Actors = [simulationLogActors; addedRogueActors];

== matlab function mOvertakeManeuver/Smart Actor/Smart Actor system/Find center of my right lane/Get right lane center Y ==
  data: currPose input; rightLaneY output; numLanes parameter
function rightLaneY = getRightLaneY(currPose, numLanes)
% Get the Y-Coordinate of the right lane center

laneBoundaries = zeros(1, numLanes + 1);
% Getting the key corresponding to the actorId from data-table
key = getScenarioTableEntryKey(uint32(1), currPose.ActorID);
completeLaneBoundaryInfo = getScenarioTableEntry(key);
for i = 1 : size(laneBoundaries, 2)
    laneBoundaries(1, i) = completeLaneBoundaryInfo.coordinates(i, 2);
end
index = 0;
% Search the right lane based on the current position
for i = 1 : size(laneBoundaries, 2) - 1
    if (currPose.Position(2) <= laneBoundaries(1, i) && currPose.Position(2) >= laneBoundaries(1, (i + 1)))
        index = i;
        break;
    end
end
if (index >= 1)
    rightLaneY = (laneBoundaries(1, index + 1) + laneBoundaries(1, (index + 2))) / 2;
else
    % No right Lane present
    rightLaneY = realmax('double');
end

== matlab function mOvertakeManeuver/Smart Actor/Smart Actor system/Get vehicles ahead in left lane/Get vehicles ahead in left lane ==
  data: currPose input; vehAheadInfo output Bus: Vehicle size=maxVehicles; numVeh output; maxVehicles parameter
function [vehAheadInfo, numVeh]  = getVehAheadLeftLaneSorted(currPose, maxVehicles)
% Call the data-table query for getting the list of vehicles ahead in
% lane left of the smart actor's lane and return the sorted list of those vehicles in increasing order of their
% distance from smart-vehicle.

actorStruct = struct('ActorID', 0, 'Position', [0 0 0], ...
    'Velocity', [0 0 0], 'Roll', 0, 'Pitch', 0, 'Yaw', 0, ...
    'AngularVelocity', [0 0 0]);
vehAheadInfo = repmat(actorStruct, maxVehicles, 1);
qHdl = initActorQueryIterator(currPose.ActorID, uint32(OvertakeQueries.VehiclesAheadLeftLane));
[key, done] = getActorQueryIterNextKey(qHdl);
mIdx = 1;
% Get next vehicle-of-interest and put in a sorted way according to its
% distance from smart-vehicle
while ~done
    info = getActorTableEntry(key);
    if(mIdx == 1) % First vehicle
        vehAheadInfo(mIdx) = info;
    else
        i = (mIdx - 1);
        gap = abs(info.Position(1) - currPose.Position(1));
        % Insert at correct place to maintain sorted order
        while(i >= 1 && (gap < abs(vehAheadInfo(i).Position(1) - currPose.Position(1))))
            vehAheadInfo(i + 1) = vehAheadInfo(i);
            i = i - 1;
        end
        vehAheadInfo(i + 1) = info;
    end
    mIdx = mIdx + 1;
    [key, done] = getActorQueryIterNextKey(qHdl);
end
numVeh = mIdx - 1;
end

== matlab function mOvertakeManeuver/Smart Actor/Smart Actor system/Get vehicles ahead in my lane/Get vehicles ahead in my lane ==
  data: currPose input; vehAheadInfo output Bus: Vehicle size=maxVehicles; numVeh output; maxVehicles parameter
function [vehAheadInfo, numVeh]  = getVehAheadSameLaneSorted(currPose, maxVehicles)
% Call the data-table query for getting the list of vehicles ahead in smart
% actor's lane and returns the sorted list of those vehicles in increasing
% order of their distance from it.

actorStruct = struct('ActorID', 0, 'Position', [0 0 0], ...
    'Velocity', [0 0 0], 'Roll', 0, 'Pitch', 0, 'Yaw', 0, ...
    'AngularVelocity', [0 0 0]);
vehAheadInfo = repmat(actorStruct, maxVehicles, 1);
qHdl = initActorQueryIterator(currPose.ActorID, uint32(OvertakeQueries.VehiclesAheadSameLane));
[key, done] = getActorQueryIterNextKey(qHdl);
mIdx = 1;
% Get next vehicle-of-interest and insert in a sorted way in order of its
% distance from smart-vehicle.
while ~done
    info = getActorTableEntry(key);
    if(mIdx == 1) % First vehicle
        vehAheadInfo(mIdx) = info;
    else
        i = (mIdx - 1);
        gap = abs(info.Position(1) - currPose.Position(1));
         % Insert at correct place to maintain sorted order
        while(i >= 1 && (gap < abs(vehAheadInfo(i).Position(1) - currPose.Position(1))))
            vehAheadInfo(i + 1) = vehAheadInfo(i);
            i = i - 1;
        end
        vehAheadInfo(i + 1) = info;
    end
    mIdx = mIdx + 1;
    [key, done] = getActorQueryIterNextKey(qHdl);
end
numVeh = mIdx - 1;
end

== matlab function mOvertakeManeuver/Smart Actor/Smart Actor system/Planner/Extract vehicle ahead info ==
  data: leadVehicleGap output; leadVehicleRelVelocity output; currPose input; maxVelocity parameter; smartActorVel output; safeTimeGap parameter; standStillGap parameter
function [leadVehicleGap, leadVehicleRelVelocity, smartActorVel] = getVehAheadInfo( ...
    currPose, maxVelocity, safeTimeGap, standStillGap)
% Get Lead vehicle info for Adaptive cruise control mode.

smartActorVel = currPose.Velocity(1);
[numVeh, vehAheadInfo] = getVehAheadSameLaneSorted(currPose);
for i=1:numVeh % Convert to self-centered pose
    vehAheadInfo(i) = globalToSelfCentered(currPose, vehAheadInfo(i));
end
if(numVeh > 0) % If there is a vehicle ahead
    leadVehicleGap = vehAheadInfo(1).Position(1);
    leadVehicleRelVelocity = vehAheadInfo(1).Velocity(1);
else
    % Set to max sensing range to give an impression that there is no
    % vehicle ahead and hence smart actor can go full throttle.
    leadVehicleGap = safeTimeGap * maxVelocity + standStillGap;
    leadVehicleRelVelocity = 0;
end

== matlab function mOvertakeManeuver/Smart Actor/Smart Actor system/Plant/Smart actor movement ==
  data: commandAccel input; commandAngle input; initPose input; updatedPose output Bus: Vehicle
function updatedPose  = simulateMovement(commandAccel, commandAngle, initPose)
% Update the position of smart vehicle based on controller outputs (command
% angle and command acceleration)

persistent actorPose;
persistent prevCommandAngle;
persistent initVelocityX;
persistent initPositionX;
persistent initVelocityY;
persistent initPositionY;
if isempty(actorPose)
    actorPose = initPose;
    prevCommandAngle = 0;
    initVelocityX = initPose.Velocity(1);
    initPositionX = initPose.Position(1);
    initVelocityY = initPose.Velocity(2);
    initPositionY = initPose.Position(2);
end

speed =  sqrt(actorPose.Velocity(1) * actorPose.Velocity(1) + actorPose.Velocity(2) * actorPose.Velocity(2));

if actorPose.Velocity(1) <= 0 && commandAccel < 0 % To avoid backward movement
    commandAccel = 0;
    actorPose.Velocity(1) = 0;
    [actorPose.Position(1), actorPose.Velocity(1)] = currentPositionX(...
        commandAccel * cosd(commandAngle), 1, actorPose.Velocity(1), actorPose.Position(1)); % For x-dir
    [actorPose.Position(2), actorPose.Velocity(2)] = currentPositionY(...
        commandAccel * sind(commandAngle), 1, actorPose.Velocity(2), actorPose.Position(2)); % For y-dir
    initPositionX = actorPose.Position(1);
    initPositionY = actorPose.Position(2);
    initVelocityX = actorPose.Velocity(1);
    initVelocityY = actorPose.Velocity(2);
else
    if(commandAngle == prevCommandAngle)
        [actorPose.Position(1), actorPose.Velocity(1)] = currentPositionX(...
            commandAccel * cosd(commandAngle), 0, initVelocityX, initPositionX); % For x-dir
        [actorPose.Position(2), actorPose.Velocity(2)] = currentPositionY(...
            commandAccel * sind(commandAngle), 0, initVelocityY, initPositionY); % For y-dir
    else
        % When direction changes, reset the two integrator blocks and set current value as initial value.
        initVelocityX = speed * cosd(commandAngle);
        initVelocityY = speed * sind(commandAngle);
        [actorPose.Position(1), actorPose.Velocity(1)] = currentPositionX(...
            commandAccel * cosd(commandAngle), 1, initVelocityX, actorPose.Position(1)); % For x-dir
        [actorPose.Position(2), actorPose.Velocity(2)] = currentPositionY(...
            commandAccel * sind(commandAngle), 1, initVelocityY, actorPose.Position(2)); % For y-dir
        initPositionX = actorPose.Position(1);
        initPositionY = actorPose.Position(2);
    end
end

prevCommandAngle = commandAngle;
updatedPose = actorPose;

== matlab function mOvertakeManeuver/Added Rogue Actors/Get initial poses ==
  data: xAcceleration output double; xVelocity output double; xPosition output; yAcceleration output; yVelocity output double; numAddedRogueActors parameter; yPosition output; initXPos parameter; initXVel parameter; initYPosRogue parameter
function [xAcceleration,xVelocity, xPosition, yAcceleration, yVelocity, yPosition] = loadInitPose(numAddedRogueActors,initXPos, initXVel, initYPosRogue)
% Output initial Rogue pose
persistent flag;
persistent xPos;
persistent yPos;
persistent xVel;
persistent yVel;
persistent xAccel;
persistent yAccel;
if(isempty(flag))
    flag = false;
    xAccel = zeros(numAddedRogueActors,1);
    yAccel = zeros(numAddedRogueActors,1);
    xPos = zeros(numAddedRogueActors,1);
    yPos = zeros(numAddedRogueActors,1);
    xVel = zeros(numAddedRogueActors,1);
    yVel = zeros(numAddedRogueActors,1);
    for i=1:numAddedRogueActors
        xPos(i) = initXPos(i);
        yPos(i) = initYPosRogue;
        xVel(i) = initXVel(i);
        yVel(i) = 0;
    end
end
xVelocity = xVel;
yVelocity = yVel;
xPosition = xPos;
yPosition = yPos;
xAcceleration = xAccel;
yAcceleration = yAccel;
end

== matlab function mOvertakeManeuver/Added Rogue Actors/Publish to data-table ==
  data: rogueActorIdBase parameter; numAddedRogueActors parameter; xVelVector input; xPosVector input; yVelVector input; yPosVector input
function PublishPose(rogueActorIdBase,numAddedRogueActors, xVelVector, ...
    xPosVector, yVelVector, yPosVector)
% Update the Pose value of the actors

actorInfo = struct('ActorID', 0, 'Position', [0 0 0], ...
    'Velocity', [0 0 0], 'Roll', 0, 'Pitch', 0, 'Yaw', 0, ...
    'AngularVelocity', [0 0 0]);
for i=1:numAddedRogueActors
    actorInfo.ActorID = rogueActorIdBase + i;
    actorInfo.Position = [xPosVector(i) yPosVector(i) 0];
    actorInfo.Velocity = [xVelVector(i) yVelVector(i) 0];
    setActorTableEntry(actorInfo.ActorID, actorInfo);
end

== matlab function mOvertakeManeuver/Smart Actor/Smart Actor system/Planner/Plan Caller ==
  data: currPose input; commandAccel output; commandAngle output; ACCTrigger output
function [commandAccel, commandAngle, ACCTrigger]  = planSelectAndExecute(currPose)
% Execute the current plan and select a new plan to execute if current plan
% has completed.

persistent planId;
persistent planStatus;
commandAngle = 0;
commandAccel = 0;
ACCTrigger = 0;
if isempty(planStatus)
    % no plan is selected
    planId = 0;
    planStatus = 0;
end

% If no plan is runnning/some plan has completed
if(planStatus == 0)
    planId = selectNewPlan(currPose);
end
% Execute the plan (either newly selected or ongoing)
if(planId > 0)
    [commandAccel, ~, commandAngle, planStatus, ACCTrigger] = ...
        evaluatePlan(planId, 1, currPose);
else
    % No plan now. Reset the plan status.
    planStatus = 0;
end
